simulink model "equalcombining"  (R2019b)
settings: Solver=VariableStepAuto  StartTime=0.0  StopTime=1  RelTol=1e-3
model workspace (MAT data in the model file):
  polarangle = 45
  snr = 100
libraries: commdigbbndfm2 x3, commchan3 x2, commrflib2 x2, commsink2 x1, commrandsrc3 x1
settings Model: Creator=William Barnhart  LastModifiedBy=William Barnhart

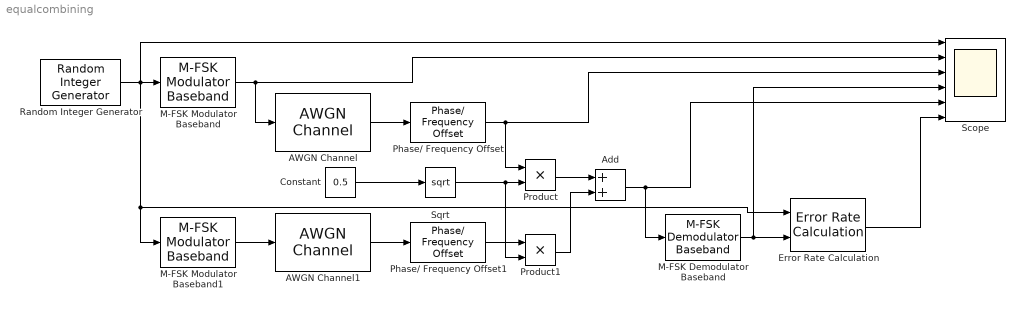
== system equalcombining ==
  AWGN Channel : commchan3/AWGN Channel  InputProcessing=Columns as channels (frame based)  seed=67  noiseMode="Signal to noise ratio  (Eb/No)"  EbNodB=snr  EsNodB=10  SNRdB=10  bitsPerSym=1  Ps=1  Tsym=0.1  variance=1
      settings: SourceProductName=Communications Toolbox
  AWGN Channel1 : commchan3/AWGN Channel  InputProcessing=Columns as channels (frame based)  seed=67  noiseMode="Signal to noise ratio  (Eb/No)"  EbNodB=snr  EsNodB=10  SNRdB=10  bitsPerSym=1  Ps=1  Tsym=0.1  variance=1
      settings: SourceProductName=Communications Toolbox
  Add : Sum
  Constant : Constant  Value=0.5
  Error Rate Calculation : commsink2/Error Rate Calculation  N=0  st_delay=0  cp_mode=Entire frame  subframe=[]  PMode=Port  WsName=ErrorVec  RsMode2=off  stop=off  numErr=100  maxBits=1e6
      settings: SourceProductName=Communications Toolbox
  M-FSK Demodulator Baseband : commdigbbndfm2/M-FSK Demodulator Baseband  M=2  OutType=Bit  Dec=Gray  freqSep=6  numSamp=17  RateOptions=Allow multirate processing  outDataType=boolean
      settings: SourceProductName=Communications Toolbox  SourceProductBaseCode=CM
  M-FSK Modulator Baseband : commdigbbndfm2/M-FSK Modulator Baseband  M=2  InType=Bit  Enc=Gray  freqSep=1000  phaseType=Discontinuous  numSamp=17  RateOptions=Allow multirate processing  outDataType=double
      settings: SourceProductName=Communications Toolbox
  M-FSK Modulator Baseband1 : commdigbbndfm2/M-FSK Modulator Baseband  M=2  InType=Bit  Enc=Gray  freqSep=1000  phaseType=Discontinuous  numSamp=17  RateOptions=Allow multirate processing  outDataType=double
      settings: SourceProductName=Communications Toolbox
  Phase/ Frequency Offset : commrflib2/Phase// Frequency Offset  phaseOffset=polarangle  freqPort=off  freqOffset=0
      settings: SourceProductName=Communications Toolbox
  Phase/ Frequency Offset1 : commrflib2/Phase// Frequency Offset  phaseOffset=90-polarangle  freqPort=off  freqOffset=0
      settings: SourceProductName=Communications Toolbox
  Product : Product
  Product1 : Product
  Random Integer Generator : commrandsrc3/Random Integer Generator  SetSize=2  SeedSource=Auto  Seed=0  SampleTime=0.1  SamplesPerFrame=1  OutputDataType=boolean  SimulateUsing=Interpreted execution
      settings: SourceProductName=Communications Toolbox
  Scope : Scope  NumInputPorts=6
  Sqrt : Sqrt  SaturateOnIntegerOverflow=on
  wires:
  Random Integer Generator/1 -> M-FSK Modulator Baseband1/1, Error Rate Calculation/1, M-FSK Modulator Baseband/1, Scope/1
  Error Rate Calculation/1 -> Scope/6
  AWGN Channel/1 -> Phase/ Frequency Offset/1
  Product1/1 -> Add/2
  M-FSK Demodulator Baseband/1 -> Error Rate Calculation/2, Scope/4
  Product/1 -> Add/1
  Constant/1 -> Sqrt/1
  M-FSK Modulator Baseband/1 -> Scope/2, AWGN Channel/1
  Phase/ Frequency Offset1/1 -> Product1/1
  AWGN Channel1/1 -> Phase/ Frequency Offset1/1
  M-FSK Modulator Baseband1/1 -> AWGN Channel1/1
  Sqrt/1 -> Product/2, Product1/2
  Phase/ Frequency Offset/1 -> Scope/3, Product/1
  Add/1 -> Scope/5, M-FSK Demodulator Baseband/1
